simulink library "FlexBeamElement_MS2G_Lib"  (R2016a)
settings: Solver=ode45  StartTime=0.0  StopTime=10.0  RelTol=1e-3
undefined symbols (not defined in the file): b, beam_length, beam_wall, beam_width, bending_stiffness, Damping, density, Extr_Data_Box, kbendingx, kbendingy, kelongz, ktwistz, matDamping, num_elem, numelem, rho, shearM, X, Y, youngsM, Z
libraries: sm_lib x335, nesl_utility x64, FlexBeamElement_MS2G_Lib x1
(part 1 of 10)
Description:
  | Copyright 2014-2016 The MathWorks, Inc.
settings Model: Creator=psanghvi  LastModifiedBy=smiller
settings DataIOCC: LimitDataPoints=on  SaveFormat=Array  SignalLoggingSaveFormat=ModelDataLogs
settings DebuggingCC: UnderspecifiedInitializationDetection=Classic  MergeDetectMultiDrivingBlocksExec=none  SolverPrmCheckMsg=warning  MultiTaskDSMMsg=warning  MultiTaskCondExecSysMsg=none  AllowSymbolicDim=off
settings HardwareCC: ProdBitPerPointer=32  ProdLargestAtomicFloat=None  ProdIntDivRoundTo=Undefined  ProdEndianess=Unspecified  ProdWordSize=32  ProdHWDeviceType=32-bit Generic
settings ModelReferenceCC: PropagateSignalLabelsOutOfModel=off
settings ConfigComp: CovModelRefEnable=Off  CovSFcnEnable=off

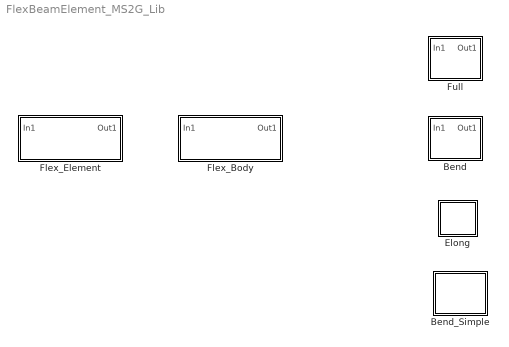
== system FlexBeamElement_MS2G_Lib ==
  Bend : Subsystem  mask{length=length, rho=rho, beam_width=beam_width, beam_wall=beam_wall, kbendingx=kbendingx, kbendingy=kbendingy, kbendingz=ktwistz, kelongz=kelongz, b=b}
      mask prompts: length "Beam Length (m)"; rho "Material Density (kg/(m^3)"; beam_width "Beam Width & Height (m)"; beam_wall "Beam Wall Thickness (m)"; kbendingx "Bending Spring Constant about X(Nm/rad)"; kbendingy "Bending Spring Constant about Y(Nm/rad)"; kbendingz "Twist Spring Constant about Z(Nm/rad)"; kelongz "Elongation Spring Constant about Z(N/m)"; b "Damping Constant (Nm/rad.s)"
  Bend_Simple : Subsystem  mask{length=length, rho=rho, beam_width=beam_width, beam_wall=beam_wall, kbendingx=kbendingx, kbendingy=kbendingy, kbendingz=ktwistz, kelongz=kelongz, b=b}
      mask prompts: length "Beam Length (m)"; rho "Material Density (kg/(m^3)"; beam_width "Beam Width & Height (m)"; beam_wall "Beam Wall Thickness (m)"; kbendingx "Bending Spring Constant about X(Nm/rad)"; kbendingy "Bending Spring Constant about Y(Nm/rad)"; kbendingz "Twist Spring Constant about Z(Nm/rad)"; kelongz "Elongation Spring Constant about Z(N/m)"; b "Damping Constant (Nm/rad.s)"
  Elong : Subsystem  mask{length=beam_length, kBending=bending_stiffness, matDamping=matDamping, beam_width=beam_width, beam_wall=beam_wall, rho=density}
      mask prompts: length "Beam Length (m)"; kBending "Bending Stiffness (N*m/rad)"; matDamping "Material Damping (N*m/(rad/s))"; beam_width "Beam Width & Height (m)"; beam_wall "Beam Wall Thickness(m)"; rho "Material Density (kg/(m^3)"
  Flex_Body : Subsystem  mask(Flexible Body){rho=density, youngsM=youngsM, shearM=shearM, numelem=num_elem, beam_length=beam_length, beam_width=beam_width, beam_wall=beam_wall, b=Damping}
      mask prompts: rho "Material Density (kg/(m^3)"; youngsM "Modulus of Elasticity (N/m2)"; shearM "Shear Modulus (N/m2)"; numelem "Number of elements"; beam_length "Beam Length (m)"; beam_width "Beam Width & Height (m)"; beam_wall "Beam Wall Thickness(m)"; b "Damping Constant (Nm/rad.s)"
      mask help:
      | Models a flexible hollow square beam based on lumped parameter method.
      | Number of flexible elements, material properties as well as beam
      | dimension can be varied from mask parameters.
      mask init:
      | [kbendingx, kbendingy, ktwistz, kelongz, length] = Compute_GFE_Prop(rho, youngsM, shearM, numelem, beam_length, beam_width,beam_wall);
      | thisblock = gcb;
      | anno = ['No of Elem: ' num2str(numelem)];
      | set_param(thisblock, 'AttributesFormatString',anno);
      | set_param([thisblock '/Matrix Concatenate'],'NumInputs','numelem')
      | blkchoice = get_param('FlexBeamElement_MS2G_Lib/Flex_Element','BlockChoice');
      | if numelem <1
      |     error('Number of Flexible elements should be greater than 0')
      | end
      | prev_flex_bod = find_system(gcb,'LookUnderMasks','all','RegExp','on','Name','Flex_Elem_*');
      | if ~isempty(prev_flex_bod)
      |     delete_block(prev_flex_bod(1:end))
      | end
      | linehan = find_system(thisblock,'LookUnderMasks','all','FindAll','on','type','line');
      | if ~isempty(linehan)
      |     delete_line(linehan)
      | end
      | blk_or = [100 155 140 195];
      | set_param([thisblock '/B'],'Position',blk_or)
      | set_param([thisblock '/' sprintf('Transform\nBeamX')],'Position',blk_or+[80 0 80 0])
      | add_line(thisblock,['B/Rconn1'],[sprintf('Transform\nBeamX') '/Lconn1'],'autorouting','on');
      | add_block('FlexBeamElement_MS2G_Lib/Flex_Element',[thisblock '/Flex_Elem_' num2str(1)],'Position',blk_or+[80 0 80 0]*2)
      | add_line(thisblock,[sprintf('Transform\nBeamX') '/Rconn1'],['Flex_Elem_' num2str(1) '/Lconn1'],'autorouting','on');
      | add_line(thisblock,'In1/1',['Flex_Elem_' num2str(1) '/1'],'autorouting','on')
      | add_line(thisblock,['Flex_Elem_' num2str(1) '/1'],'Matrix Concatenate/1','autorouting','on')
      | set_param([thisblock '/Flex_Elem_' num2str(1)], 'LinkStatus', 'none')
      | set_param([thisblock '/Flex_Elem_' num2str(1) '/' blkchoice], 'LinkStatus', 'none')
      | set_param([thisblock '/Flex_Elem_' num2str(1) '/' blkchoice '/Selector'],'InputPortWidth','3*numelem')
      | set_param([thisblock '/Flex_Elem_' num2str(1) '/' blkchoice '/Selector'],'Indices','[1 2 3]')
      | if strcmp(blkchoice,'Full')
      |     state_order{1} = [thisblock '/Flex_Elem_' num2str(1) '/' blkchoice '/Bearing Joint'];
      | elseif strcmp(blkchoice,'Elong')
      |     state_order{1} = [thisblock '/Flex_Elem_' num2str(1) '/' blkchoice '/Prismatic Joint'];
      | else
      |     state_order{1} = [thisblock '/Flex_Elem_' num2str(1) '/' blkchoice '/Revolute Joint'];
      | end
      | for i = 2:1:numelem
      |     add_block('FlexBeamElement_MS2G_Lib/Flex_Element',[thisblock '/Flex_Elem_' num2str(i)],'Position',blk_or+(i+1)*[80 0 80 0])
      |     add_line(thisblock,['Flex_Elem_' num2str(i-1) '/Rconn1'],['Flex_Elem_' num2str(i) '/Lconn1'],'autorouting','on');
      |     add_line(thisblock,'In1/1',['Flex_Elem_' num2str(i) '/1'],'autorouting','on')
      |     add_line(thisblock,['Flex_Elem_' num2str(i) '/1'],['Matrix Concatenate/' num2str(i)],'autorouting','on')
      |     set_param([thisblock '/Flex_Elem_' num2str(i)], 'LinkStatus', 'none')
      |     set_param([thisblock '/Flex_Elem_' num2str(i) '/' blkchoice], 'LinkStatus', 'none')
      |     set_param([thisblock '/Flex_Elem_' num2str(i) '/' blkchoice '/Selector'],'InputPortWidth','3*numelem')
      |     set_param([thisblock '/Flex_Elem_' num2str(i) '/' blkchoice '/Selector'],'Indices',['[' num2str([3*i-2 3*i-1 3*i]) ']'])
      |     if strcmp(blkchoice,'Full')
      |         state_order{i} = [thisblock '/Flex_Elem_' num2str(i) '/' blkchoice '/Bearing Joint'];
      |     elseif strcmp(blkchoice,'Elong')
      |         state_order{i} = [thisblock '/Flex_Elem_' num2str(i) '/' blkchoice '/Prismatic Joint'];
      |     else
      |         state_order{i} = [thisblock '/Flex_Elem_' num2str(i) '/' blkchoice '/Revolute Joint'];
      |     end
      | end
      | set_param([thisblock '/F'],'Position',blk_or+ (numelem+2)*[80 0 80 0]);
      | add_line(thisblock,['Flex_Elem_' num2str(numelem) '/Rconn1'],['F/Rconn1'],'autorouting','on');
      | assignin('base','State_order',state_order)
      | add_line(thisblock,'Matrix Concatenate/1','Out1/1','autorouting','on')
      settings: AttributesFormatString=No of Elem: 30  CopyFcn=set_param(gcb, 'LinkStatus', 'none')
      mask Display:
      | image(imread('Flexible_Beam.png'));
      | port_label('input',1,'F_L');
      | port_label('output',1,'wz');
      | color red
      | port_label('LConn',1,'B');
      | port_label('RConn',1,'F');
  Flex_Element : Subsystem  BlockChoice=Full
      settings: TemplateBlock=self  MemberBlocks=Bend,Elong,Full
  Full : Subsystem  mask{length=length, rho=rho, beam_width=beam_width, beam_wall=beam_wall, kbendingx=kbendingx, kbendingy=kbendingy, kbendingz=ktwistz, kelongz=kelongz, b=b}
      mask prompts: length "Beam Length (m)"; rho "Material Density (kg/(m^3)"; beam_width "Beam Width & Height (m)"; beam_wall "Beam Wall Thickness (m)"; kbendingx "Bending Spring Constant about X(Nm/rad)"; kbendingy "Bending Spring Constant about Y(Nm/rad)"; kbendingz "Twist Spring Constant about Z(Nm/rad)"; kelongz "Elongation Spring Constant about Z(N/m)"; b "Damping Constant (Nm/rad.s)"

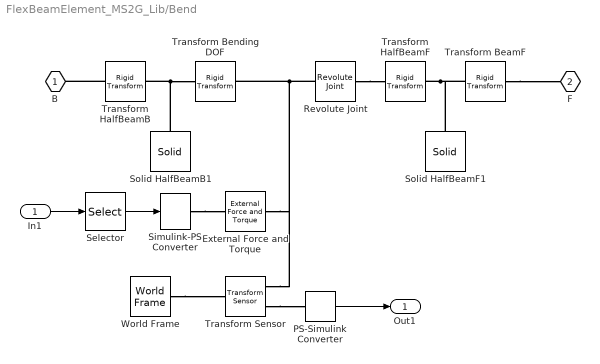
== system FlexBeamElement_MS2G_Lib/Bend ==
  In1 : Inport
  " Transform Bending DOF" : sm_lib/Frames and Transforms/Rigid Transform  TranslationMethod=StandardAxis  TranslationLengthUnit=m  TranslationStandardAxis=+Z  TranslationStandardOffset=length/4  TranslationCartesianOffset=[0 0 0]  TranslationROffset=0  TranslationROffsetUnits=m  TranslationZOffset=0  TranslationZOffsetUnits=m  TranslationThetaOffset=0  TranslationThetaOffsetUnits=deg  RotationMethod=StandardAxis  RotationAngleUnits=deg  RotationStandardAxis=+Y  RotationAngle=90  RotationArbitraryAxis=[0 0 1]  FollAlignAxisA=+X  BaseAlignAxisA=+Y  FollAlignAxisB=+Y  BaseAlignAxisB=+Z  RotationSequenceAxes=FollowerAxes  RotationSequence=XYX  RotationSequenceAngles=[0 0 0]  RotationSequenceAnglesUnits=deg  RotationMatrix=[1 0 0; 0 1 0; 0 0 1]
  " Transform BeamF" : sm_lib/Frames and Transforms/Rigid Transform  TranslationMethod=StandardAxis  TranslationLengthUnit=m  TranslationStandardAxis=+Z  TranslationStandardOffset=length/4  TranslationCartesianOffset=[0 0 0]  TranslationROffset=0  TranslationROffsetUnits=m  TranslationZOffset=0  TranslationZOffsetUnits=m  TranslationThetaOffset=0  TranslationThetaOffsetUnits=deg  RotationMethod=None  RotationAngleUnits=deg  RotationStandardAxis=+Z  RotationAngle=0  RotationArbitraryAxis=[0 0 1]  FollAlignAxisA=+X  BaseAlignAxisA=+Y  FollAlignAxisB=+Y  BaseAlignAxisB=+Z  RotationSequenceAxes=FollowerAxes  RotationSequence=XYX  RotationSequenceAngles=[0 0 0]  RotationSequenceAnglesUnits=deg  RotationMatrix=[1 0 0; 0 1 0; 0 0 1]
  External Force and Torque : sm_lib/Forces and Torques/External Force and Torque  ForceResolutionFrame=AttachedFrame  EnableForceX=off  EnableForceY=off  EnableForceZ=off  EnableForce=on  TorqueResolutionFrame=AttachedFrame  EnableTorqueX=off  EnableTorqueY=off  EnableTorqueZ=off  EnableTorque=off
  PS-Simulink Converter : nesl_utility/PS-Simulink Converter  PhysicalDomain=network_engine_domain  SubClassName=ps_output  LeftPortType=input  RightPortType=output  PseudoPeriodic=off  Frequencies=[]  Unit=1  AffineConversion=off
  Revolute Joint : sm_lib/Joints/Revolute Joint  SenseConstraintForce=off  SenseConstraintForceX=off  SenseConstraintForceY=off  SenseConstraintForceZ=off  SenseConstraintTorque=off  SenseConstraintTorqueX=off  SenseConstraintTorqueY=off  SenseConstraintTorqueZ=off  SenseTotalForce=off  SenseTotalForceX=off  SenseTotalForceY=off  SenseTotalForceZ=off  SenseTotalTorque=off  SenseTotalTorqueX=off  SenseTotalTorqueY=off  SenseTotalTorqueZ=off  CompositeWrenchDir=FollowerOnBase  CompositeWrenchFrame=BaseFrame  EquilibriumPosition=0  EquilibriumPositionUnits=deg  SpringStiffness=kbendingx  SpringStiffnessUnits=N*m/rad  DampingCoefficient=b  DampingCoefficientUnits=N*m/(rad/s)  TorqueActuationMode=NoTorque  MotionActuationMode=ComputedMotion  SensePosition=off  SenseVelocity=off  SenseAcceleration=off  SenseTorqueForce=off  PositionTargetSpecify=off  PositionTargetPriority=High  PositionTargetValue=0  PositionTargetValueUnits=deg  VelocityTargetSpecify=off  VelocityTargetPriority=High  VelocityTargetValue=0  VelocityTargetValueUnits=deg/s
  Selector : Selector  InputPortWidth=numelem*3  IndexOptions=Index vector (dialog)  Indices=[1 3]  OutputSizes=1
  Simulink-PS Converter : nesl_utility/Simulink-PS Converter  PhysicalDomain=network_engine_domain  SubClassName=ps_input  LeftPortType=input  RightPortType=output  PseudoPeriodic=off  Frequencies=[]  NoiseDistribution=none  NoiseParameters=[]  Unit=1  AffineConversion=off  InputFiltering=off  SimscapeFilterOrder=1  InputFilterTimeConstant=0.001  UdotUserProvided=1
  Solid HalfBeamB1 : sm_lib/Body Elements/Solid  InertiaType=CalculateFromGeometry  Mass=1  MassUnits=kg  CenterOfMass=[0 0 0]  CenterOfMassUnits=m  MomentsOfInertia=[1 1 1]  MomentsOfInertiaUnits=kg*m^2  ProductsOfInertia=[0 0 0]  ProductsOfInertiaUnits=kg*m^2  DensityBased=on  Density=rho  DensityUnits=kg/(m^3)  DoExposeReferenceFrame=on  SerializedFrames=<Frames/>  GraphicType=FromGeometry  MarkerShape=Sphere  MarkerSize=10  MarkerSizeUnits=m  GraphicVisPropType=SimpleVisualProperties  GraphicDiffuseColor=[0.5 0.5 0.5]  GraphicSpecularColor=[0.5 0.5 0.5 1.0]  GraphicAmbientColor=[0.15 0.15 0.15 1.0]  GraphicEmissiveColor=[0.0 0.0 0.0 1.0]  GraphicShininess=75  GraphicOpacity=1.0  GeometryShape=GeneralExtrusion  RectangleSize=[1 1]  RectangleSizeUnits=m  BrickDimensions=[1 1 1]  BrickDimensionUnits=m  CylinderRadius=1  CylinderRadiusUnits=m  CylinderLength=1  CylinderLengthUnits=m  SphereRadius=1  SphereRadiusUnits=m  EllipsoidRadii=[1 1 1]  EllipsoidRadiiUnits=m  ExtrusionCrossSection=Extr_Data_Box(beam_width,beam_width-2*beam_wall,beam_width,beam_width-2*beam_wall)  ExtrusionCrossSectionUnits=m  ExtrusionLength=length/2  ExtrusionLengthUnits=m  PolygonNumSides=3  PolygonOuterRadius=1  PolygonOuterRadiusUnits=m  ExtGeomFileType=STL  ExtGeomFileUnits=m  RevolutionCrossSection=[1 1; 1 -1; 2 -1; 2 1]  RevolutionCrossSectionUnits=m  RevolutionExtent=Full  RevolutionAngle=180  RevolutionAngleUnits=deg
  Solid HalfBeamF1 : sm_lib/Body Elements/Solid  InertiaType=CalculateFromGeometry  Mass=1  MassUnits=kg  CenterOfMass=[0 0 0]  CenterOfMassUnits=m  MomentsOfInertia=[1 1 1]  MomentsOfInertiaUnits=kg*m^2  ProductsOfInertia=[0 0 0]  ProductsOfInertiaUnits=kg*m^2  DensityBased=on  Density=rho  DensityUnits=kg/(m^3)  DoExposeReferenceFrame=on  SerializedFrames=<Frames/>  GraphicType=FromGeometry  MarkerShape=Sphere  MarkerSize=10  MarkerSizeUnits=m  GraphicVisPropType=SimpleVisualProperties  GraphicDiffuseColor=[0.5 0.5 0.5]  GraphicSpecularColor=[0.5 0.5 0.5 1.0]  GraphicAmbientColor=[0.15 0.15 0.15 1.0]  GraphicEmissiveColor=[0.0 0.0 0.0 1.0]  GraphicShininess=75  GraphicOpacity=1.0  GeometryShape=GeneralExtrusion  RectangleSize=[1 1]  RectangleSizeUnits=m  BrickDimensions=[1 1 1]  BrickDimensionUnits=m  CylinderRadius=1  CylinderRadiusUnits=m  CylinderLength=1  CylinderLengthUnits=m  SphereRadius=1  SphereRadiusUnits=m  EllipsoidRadii=[1 1 1]  EllipsoidRadiiUnits=m  ExtrusionCrossSection=Extr_Data_Box(beam_width,beam_width-2*beam_wall,beam_width,beam_width-2*beam_wall)  ExtrusionCrossSectionUnits=m  ExtrusionLength=length/2  ExtrusionLengthUnits=m  PolygonNumSides=3  PolygonOuterRadius=1  PolygonOuterRadiusUnits=m  ExtGeomFileType=STL  ExtGeomFileUnits=m  RevolutionCrossSection=[1 1; 1 -1; 2 -1; 2 1]  RevolutionCrossSectionUnits=m  RevolutionExtent=Full  RevolutionAngle=180  RevolutionAngleUnits=deg
  Transform HalfBeamB : sm_lib/Frames and Transforms/Rigid Transform  TranslationMethod=StandardAxis  TranslationLengthUnit=m  TranslationStandardAxis=+Z  TranslationStandardOffset=length/4  TranslationCartesianOffset=[0 0 0]  TranslationROffset=0  TranslationROffsetUnits=m  TranslationZOffset=0  TranslationZOffsetUnits=m  TranslationThetaOffset=0  TranslationThetaOffsetUnits=deg  RotationMethod=None  RotationAngleUnits=deg  RotationStandardAxis=+Z  RotationAngle=0  RotationArbitraryAxis=[0 0 1]  FollAlignAxisA=+X  BaseAlignAxisA=+Y  FollAlignAxisB=+Y  BaseAlignAxisB=+Z  RotationSequenceAxes=FollowerAxes  RotationSequence=XYX  RotationSequenceAngles=[0 0 0]  RotationSequenceAnglesUnits=deg  RotationMatrix=[1 0 0; 0 1 0; 0 0 1]
  Transform HalfBeamF : sm_lib/Frames and Transforms/Rigid Transform  TranslationMethod=StandardAxis  TranslationLengthUnit=m  TranslationStandardAxis=+Z  TranslationStandardOffset=-length/4  TranslationCartesianOffset=[0 0 0]  TranslationROffset=0  TranslationROffsetUnits=m  TranslationZOffset=0  TranslationZOffsetUnits=m  TranslationThetaOffset=0  TranslationThetaOffsetUnits=deg  RotationMethod=StandardAxis  RotationAngleUnits=deg  RotationStandardAxis=+Y  RotationAngle=90  RotationArbitraryAxis=[0 0 1]  FollAlignAxisA=+X  BaseAlignAxisA=+Y  FollAlignAxisB=+Y  BaseAlignAxisB=+Z  RotationSequenceAxes=FollowerAxes  RotationSequence=XYX  RotationSequenceAngles=[0 0 0]  RotationSequenceAnglesUnits=deg  RotationMatrix=[1 0 0; 0 1 0; 0 0 1]
  Transform Sensor : sm_lib/Frames and Transforms/Transform Sensor  MeasurementFrame=World  SenseAngle=off  SenseAxis=off  SenseAngle1=off  SenseAngle2=off  SenseAngle3=off  SenseQ=off  SenseR=off  SenseOmegaX=off  SenseOmegaY=off  SenseOmegaZ=on  SenseOmega1=off  SenseOmega2=off  SenseOmega3=off  SenseQDot=off  SenseRDot=off  SenseAlphaX=off  SenseAlphaY=off  SenseAlphaZ=off  SenseAlpha1=off  SenseAlpha2=off  SenseAlpha3=off  SenseQDDot=off  SenseRDDot=off  SenseX=off  SenseY=off  SenseZ=off  SenseRad=off  SenseAzim=off  SenseDist=off  SenseInc=off  SenseXDot=off  SenseYDot=off  SenseZDot=off  SenseRadDot=off  SenseAzimDot=off  SenseDistDot=off  SenseIncDot=off  SenseXDDot=off  SenseYDDot=off  SenseZDDot=off  SenseRadDDot=off  SenseAzimDDot=off  SenseDistDDot=off  SenseIncDDot=off
  World Frame : sm_lib/Frames and Transforms/World Frame
  B : PMIOPort  Port=1  Side=Left
  F : PMIOPort  Port=2  Side=Right
  Out1 : Outport
  wires:
  In1/1 -> Selector/1
  Selector/1 -> Simulink-PS Converter/1
  PS-Simulink Converter/1 -> Out1/1
  connections:
  " Transform BeamF"/RConn1 -- F/RConn1
  Transform HalfBeamB/LConn1 -- B/RConn1
  Transform HalfBeamF/LConn1 -- " Transform BeamF"/LConn1 -- Solid HalfBeamF1/RConn1
  Solid HalfBeamB1/RConn1 -- Transform HalfBeamB/RConn1 -- " Transform Bending DOF"/LConn1
  Revolute Joint/RConn1 -- Transform HalfBeamF/RConn1
  Revolute Joint/LConn1 -- Transform Sensor/RConn1 -- External Force and Torque/RConn1 -- " Transform Bending DOF"/RConn1
  Simulink-PS Converter/RConn1 -- External Force and Torque/LConn1
  World Frame/RConn1 -- Transform Sensor/LConn1
  Transform Sensor/RConn2 -- PS-Simulink Converter/LConn1

== system FlexBeamElement_MS2G_Lib/Bend_Simple ==
  " Transform BeamF" : sm_lib/Frames and Transforms/Rigid Transform  TranslationMethod=StandardAxis  TranslationLengthUnit=m  TranslationStandardAxis=+Z  TranslationStandardOffset=length/4  TranslationCartesianOffset=[0 0 0]  TranslationROffset=0  TranslationROffsetUnits=m  TranslationZOffset=0  TranslationZOffsetUnits=m  TranslationThetaOffset=0  TranslationThetaOffsetUnits=deg  RotationMethod=None  RotationAngleUnits=deg  RotationStandardAxis=+Z  RotationAngle=0  RotationArbitraryAxis=[0 0 1]  FollAlignAxisA=+X  BaseAlignAxisA=+Y  FollAlignAxisB=+Y  BaseAlignAxisB=+Z  RotationSequenceAxes=FollowerAxes  RotationSequence=XYX  RotationSequenceAngles=[0 0 0]  RotationSequenceAnglesUnits=deg  RotationMatrix=[1 0 0; 0 1 0; 0 0 1]
  " Transform Bending DOF" : sm_lib/Frames and Transforms/Rigid Transform  TranslationMethod=StandardAxis  TranslationLengthUnit=m  TranslationStandardAxis=+Z  TranslationStandardOffset=length/4  TranslationCartesianOffset=[0 0 0]  TranslationROffset=0  TranslationROffsetUnits=m  TranslationZOffset=0  TranslationZOffsetUnits=m  TranslationThetaOffset=0  TranslationThetaOffsetUnits=deg  RotationMethod=StandardAxis  RotationAngleUnits=deg  RotationStandardAxis=+Y  RotationAngle=90  RotationArbitraryAxis=[0 0 1]  FollAlignAxisA=+X  BaseAlignAxisA=+Y  FollAlignAxisB=+Y  BaseAlignAxisB=+Z  RotationSequenceAxes=FollowerAxes  RotationSequence=XYX  RotationSequenceAngles=[0 0 0]  RotationSequenceAnglesUnits=deg  RotationMatrix=[1 0 0; 0 1 0; 0 0 1]
  Revolute Joint : sm_lib/Joints/Revolute Joint  SenseConstraintForce=off  SenseConstraintForceX=off  SenseConstraintForceY=off  SenseConstraintForceZ=off  SenseConstraintTorque=off  SenseConstraintTorqueX=off  SenseConstraintTorqueY=off  SenseConstraintTorqueZ=off  SenseTotalForce=off  SenseTotalForceX=off  SenseTotalForceY=off  SenseTotalForceZ=off  SenseTotalTorque=off  SenseTotalTorqueX=off  SenseTotalTorqueY=off  SenseTotalTorqueZ=off  CompositeWrenchDir=FollowerOnBase  CompositeWrenchFrame=BaseFrame  EquilibriumPosition=0  EquilibriumPositionUnits=deg  SpringStiffness=kbendingx  SpringStiffnessUnits=N*m/rad  DampingCoefficient=b  DampingCoefficientUnits=N*m/(rad/s)  TorqueActuationMode=NoTorque  MotionActuationMode=ComputedMotion  SensePosition=off  SenseVelocity=off  SenseAcceleration=off  SenseTorqueForce=off  PositionTargetSpecify=off  PositionTargetPriority=High  PositionTargetValue=0  PositionTargetValueUnits=deg  VelocityTargetSpecify=off  VelocityTargetPriority=High  VelocityTargetValue=0  VelocityTargetValueUnits=deg/s
  Solid HalfBeamB1 : sm_lib/Body Elements/Solid  InertiaType=CalculateFromGeometry  Mass=1  MassUnits=kg  CenterOfMass=[0 0 0]  CenterOfMassUnits=m  MomentsOfInertia=[1 1 1]  MomentsOfInertiaUnits=kg*m^2  ProductsOfInertia=[0 0 0]  ProductsOfInertiaUnits=kg*m^2  DensityBased=on  Density=rho  DensityUnits=kg/(m^3)  DoExposeReferenceFrame=on  SerializedFrames=<Frames/>  GraphicType=FromGeometry  MarkerShape=Sphere  MarkerSize=10  MarkerSizeUnits=m  GraphicVisPropType=SimpleVisualProperties  GraphicDiffuseColor=[0.5 0.5 0.5]  GraphicSpecularColor=[0.5 0.5 0.5 1.0]  GraphicAmbientColor=[0.15 0.15 0.15 1.0]  GraphicEmissiveColor=[0.0 0.0 0.0 1.0]  GraphicShininess=75  GraphicOpacity=1.0  GeometryShape=GeneralExtrusion  RectangleSize=[1 1]  RectangleSizeUnits=m  BrickDimensions=[1 1 1]  BrickDimensionUnits=m  CylinderRadius=1  CylinderRadiusUnits=m  CylinderLength=1  CylinderLengthUnits=m  SphereRadius=1  SphereRadiusUnits=m  EllipsoidRadii=[1 1 1]  EllipsoidRadiiUnits=m  ExtrusionCrossSection=Extr_Data_Box(beam_width,beam_width-2*beam_wall,beam_width,beam_width-2*beam_wall)  ExtrusionCrossSectionUnits=m  ExtrusionLength=length/2  ExtrusionLengthUnits=m  PolygonNumSides=3  PolygonOuterRadius=1  PolygonOuterRadiusUnits=m  ExtGeomFileType=STL  ExtGeomFileUnits=m  RevolutionCrossSection=[1 1; 1 -1; 2 -1; 2 1]  RevolutionCrossSectionUnits=m  RevolutionExtent=Full  RevolutionAngle=180  RevolutionAngleUnits=deg
  Solid HalfBeamF1 : sm_lib/Body Elements/Solid  InertiaType=CalculateFromGeometry  Mass=1  MassUnits=kg  CenterOfMass=[0 0 0]  CenterOfMassUnits=m  MomentsOfInertia=[1 1 1]  MomentsOfInertiaUnits=kg*m^2  ProductsOfInertia=[0 0 0]  ProductsOfInertiaUnits=kg*m^2  DensityBased=on  Density=rho  DensityUnits=kg/(m^3)  DoExposeReferenceFrame=on  SerializedFrames=<Frames/>  GraphicType=FromGeometry  MarkerShape=Sphere  MarkerSize=10  MarkerSizeUnits=m  GraphicVisPropType=SimpleVisualProperties  GraphicDiffuseColor=[0.5 0.5 0.5]  GraphicSpecularColor=[0.5 0.5 0.5 1.0]  GraphicAmbientColor=[0.15 0.15 0.15 1.0]  GraphicEmissiveColor=[0.0 0.0 0.0 1.0]  GraphicShininess=75  GraphicOpacity=1.0  GeometryShape=GeneralExtrusion  RectangleSize=[1 1]  RectangleSizeUnits=m  BrickDimensions=[1 1 1]  BrickDimensionUnits=m  CylinderRadius=1  CylinderRadiusUnits=m  CylinderLength=1  CylinderLengthUnits=m  SphereRadius=1  SphereRadiusUnits=m  EllipsoidRadii=[1 1 1]  EllipsoidRadiiUnits=m  ExtrusionCrossSection=Extr_Data_Box(beam_width,beam_width-2*beam_wall,beam_width,beam_width-2*beam_wall)  ExtrusionCrossSectionUnits=m  ExtrusionLength=length/2  ExtrusionLengthUnits=m  PolygonNumSides=3  PolygonOuterRadius=1  PolygonOuterRadiusUnits=m  ExtGeomFileType=STL  ExtGeomFileUnits=m  RevolutionCrossSection=[1 1; 1 -1; 2 -1; 2 1]  RevolutionCrossSectionUnits=m  RevolutionExtent=Full  RevolutionAngle=180  RevolutionAngleUnits=deg
  Transform HalfBeamB : sm_lib/Frames and Transforms/Rigid Transform  TranslationMethod=StandardAxis  TranslationLengthUnit=m  TranslationStandardAxis=+Z  TranslationStandardOffset=length/4  TranslationCartesianOffset=[0 0 0]  TranslationROffset=0  TranslationROffsetUnits=m  TranslationZOffset=0  TranslationZOffsetUnits=m  TranslationThetaOffset=0  TranslationThetaOffsetUnits=deg  RotationMethod=None  RotationAngleUnits=deg  RotationStandardAxis=+Z  RotationAngle=0  RotationArbitraryAxis=[0 0 1]  FollAlignAxisA=+X  BaseAlignAxisA=+Y  FollAlignAxisB=+Y  BaseAlignAxisB=+Z  RotationSequenceAxes=FollowerAxes  RotationSequence=XYX  RotationSequenceAngles=[0 0 0]  RotationSequenceAnglesUnits=deg  RotationMatrix=[1 0 0; 0 1 0; 0 0 1]
  Transform HalfBeamF : sm_lib/Frames and Transforms/Rigid Transform  TranslationMethod=StandardAxis  TranslationLengthUnit=m  TranslationStandardAxis=+Z  TranslationStandardOffset=-length/4  TranslationCartesianOffset=[0 0 0]  TranslationROffset=0  TranslationROffsetUnits=m  TranslationZOffset=0  TranslationZOffsetUnits=m  TranslationThetaOffset=0  TranslationThetaOffsetUnits=deg  RotationMethod=StandardAxis  RotationAngleUnits=deg  RotationStandardAxis=+Y  RotationAngle=90  RotationArbitraryAxis=[0 0 1]  FollAlignAxisA=+X  BaseAlignAxisA=+Y  FollAlignAxisB=+Y  BaseAlignAxisB=+Z  RotationSequenceAxes=FollowerAxes  RotationSequence=XYX  RotationSequenceAngles=[0 0 0]  RotationSequenceAnglesUnits=deg  RotationMatrix=[1 0 0; 0 1 0; 0 0 1]
  B : PMIOPort  Port=1  Side=Left
  F : PMIOPort  Port=2  Side=Right
  connections:
  Revolute Joint/LConn1 -- " Transform Bending DOF"/RConn1
  Revolute Joint/RConn1 -- Transform HalfBeamF/RConn1
  " Transform Bending DOF"/LConn1 -- Transform HalfBeamB/RConn1 -- Solid HalfBeamB1/RConn1
  Solid HalfBeamF1/RConn1 -- " Transform BeamF"/LConn1 -- Transform HalfBeamF/LConn1
  Transform HalfBeamB/LConn1 -- B/RConn1
  " Transform BeamF"/RConn1 -- F/RConn1

== system FlexBeamElement_MS2G_Lib/Elong ==
  " Transform Bending DOF" : sm_lib/Frames and Transforms/Rigid Transform  TranslationMethod=StandardAxis  TranslationLengthUnit=m  TranslationStandardAxis=+Z  TranslationStandardOffset=length/4  TranslationCartesianOffset=[0 0 0]  TranslationROffset=0  TranslationROffsetUnits=m  TranslationZOffset=0  TranslationZOffsetUnits=m  TranslationThetaOffset=0  TranslationThetaOffsetUnits=deg  RotationMethod=None  RotationAngleUnits=deg  RotationStandardAxis=+Y  RotationAngle=90  RotationArbitraryAxis=[0 0 1]  FollAlignAxisA=+X  BaseAlignAxisA=+Y  FollAlignAxisB=+Y  BaseAlignAxisB=+Z  RotationSequenceAxes=FollowerAxes  RotationSequence=XYX  RotationSequenceAngles=[0 0 0]  RotationSequenceAnglesUnits=deg  RotationMatrix=[1 0 0; 0 1 0; 0 0 1]
  " Transform BeamF" : sm_lib/Frames and Transforms/Rigid Transform  TranslationMethod=StandardAxis  TranslationLengthUnit=m  TranslationStandardAxis=+Z  TranslationStandardOffset=length/4  TranslationCartesianOffset=[0 0 0]  TranslationROffset=0  TranslationROffsetUnits=m  TranslationZOffset=0  TranslationZOffsetUnits=m  TranslationThetaOffset=0  TranslationThetaOffsetUnits=deg  RotationMethod=None  RotationAngleUnits=deg  RotationStandardAxis=+Z  RotationAngle=0  RotationArbitraryAxis=[0 0 1]  FollAlignAxisA=+X  BaseAlignAxisA=+Y  FollAlignAxisB=+Y  BaseAlignAxisB=+Z  RotationSequenceAxes=FollowerAxes  RotationSequence=XYX  RotationSequenceAngles=[0 0 0]  RotationSequenceAnglesUnits=deg  RotationMatrix=[1 0 0; 0 1 0; 0 0 1]
  Prismatic Joint : sm_lib/Joints/Prismatic Joint  SenseConstraintForce=off  SenseConstraintForceX=off  SenseConstraintForceY=off  SenseConstraintForceZ=off  SenseConstraintTorque=off  SenseConstraintTorqueX=off  SenseConstraintTorqueY=off  SenseConstraintTorqueZ=off  SenseTotalForce=off  SenseTotalForceX=off  SenseTotalForceY=off  SenseTotalForceZ=off  SenseTotalTorque=off  SenseTotalTorqueX=off  SenseTotalTorqueY=off  SenseTotalTorqueZ=off  CompositeWrenchDir=FollowerOnBase  CompositeWrenchFrame=BaseFrame  EquilibriumPosition=0  EquilibriumPositionUnits=m  SpringStiffness=0  SpringStiffnessUnits=N/m  DampingCoefficient=0  DampingCoefficientUnits=N/(m/s)  TorqueActuationMode=NoTorque  MotionActuationMode=ComputedMotion  SensePosition=off  SenseVelocity=off  SenseAcceleration=off  SenseTorqueForce=off  PositionTargetSpecify=off  PositionTargetPriority=High  PositionTargetValue=0  PositionTargetValueUnits=m  VelocityTargetSpecify=off  VelocityTargetPriority=High  VelocityTargetValue=0  VelocityTargetValueUnits=m/s
  Solid HalfBeamB : sm_lib/Body Elements/Solid  InertiaType=CalculateFromGeometry  Mass=1  MassUnits=kg  CenterOfMass=[0 0 0]  CenterOfMassUnits=m  MomentsOfInertia=[1 1 1]  MomentsOfInertiaUnits=kg*m^2  ProductsOfInertia=[0 0 0]  ProductsOfInertiaUnits=kg*m^2  DensityBased=on  Density=rho  DensityUnits=kg/(m^3)  DoExposeReferenceFrame=on  SerializedFrames=<Frames/>  GraphicType=FromGeometry  MarkerShape=Sphere  MarkerSize=10  MarkerSizeUnits=m  GraphicVisPropType=SimpleVisualProperties  GraphicDiffuseColor=[0.5 0.5 0.5]  GraphicSpecularColor=[0.5 0.5 0.5 1.0]  GraphicAmbientColor=[0.15 0.15 0.15 1.0]  GraphicEmissiveColor=[0.0 0.0 0.0 1.0]  GraphicShininess=75  GraphicOpacity=1.0  GeometryShape=GeneralExtrusion  RectangleSize=[1 1]  RectangleSizeUnits=m  BrickDimensions=[1 1 1]  BrickDimensionUnits=m  CylinderRadius=1  CylinderRadiusUnits=m  CylinderLength=1  CylinderLengthUnits=m  SphereRadius=1  SphereRadiusUnits=m  EllipsoidRadii=[1 1 1]  EllipsoidRadiiUnits=m  ExtrusionCrossSection=Extr_Data_Box(beam_width,beam_width-2*beam_wall,beam_width,beam_width-2*beam_wall)  ExtrusionCrossSectionUnits=m  ExtrusionLength=length/2  ExtrusionLengthUnits=m  PolygonNumSides=3  PolygonOuterRadius=1  PolygonOuterRadiusUnits=m  ExtGeomFileType=STL  ExtGeomFileUnits=m  RevolutionCrossSection=[1 1; 1 -1; 2 -1; 2 1]  RevolutionCrossSectionUnits=m  RevolutionExtent=Full  RevolutionAngle=180  RevolutionAngleUnits=deg
  Solid HalfBeamF : sm_lib/Body Elements/Solid  InertiaType=CalculateFromGeometry  Mass=1  MassUnits=kg  CenterOfMass=[0 0 0]  CenterOfMassUnits=m  MomentsOfInertia=[1 1 1]  MomentsOfInertiaUnits=kg*m^2  ProductsOfInertia=[0 0 0]  ProductsOfInertiaUnits=kg*m^2  DensityBased=on  Density=rho  DensityUnits=kg/(m^3)  DoExposeReferenceFrame=on  SerializedFrames=<Frames/>  GraphicType=FromGeometry  MarkerShape=Sphere  MarkerSize=10  MarkerSizeUnits=m  GraphicVisPropType=SimpleVisualProperties  GraphicDiffuseColor=[0.5 0.5 0.5]  GraphicSpecularColor=[0.5 0.5 0.5 1.0]  GraphicAmbientColor=[0.15 0.15 0.15 1.0]  GraphicEmissiveColor=[0.0 0.0 0.0 1.0]  GraphicShininess=75  GraphicOpacity=1.0  GeometryShape=GeneralExtrusion  RectangleSize=[1 1]  RectangleSizeUnits=m  BrickDimensions=[1 1 1]  BrickDimensionUnits=m  CylinderRadius=1  CylinderRadiusUnits=m  CylinderLength=1  CylinderLengthUnits=m  SphereRadius=1  SphereRadiusUnits=m  EllipsoidRadii=[1 1 1]  EllipsoidRadiiUnits=m  ExtrusionCrossSection=Extr_Data_Box(beam_width,beam_width-2*beam_wall,beam_width,beam_width-2*beam_wall)  ExtrusionCrossSectionUnits=m  ExtrusionLength=length/2  ExtrusionLengthUnits=m  PolygonNumSides=3  PolygonOuterRadius=1  PolygonOuterRadiusUnits=m  ExtGeomFileType=STL  ExtGeomFileUnits=m  RevolutionCrossSection=[1 1; 1 -1; 2 -1; 2 1]  RevolutionCrossSectionUnits=m  RevolutionExtent=Full  RevolutionAngle=180  RevolutionAngleUnits=deg
  Transform HalfBeamB : sm_lib/Frames and Transforms/Rigid Transform  TranslationMethod=StandardAxis  TranslationLengthUnit=m  TranslationStandardAxis=+Z  TranslationStandardOffset=length/4  TranslationCartesianOffset=[0 0 0]  TranslationROffset=0  TranslationROffsetUnits=m  TranslationZOffset=0  TranslationZOffsetUnits=m  TranslationThetaOffset=0  TranslationThetaOffsetUnits=deg  RotationMethod=None  RotationAngleUnits=deg  RotationStandardAxis=+Z  RotationAngle=0  RotationArbitraryAxis=[0 0 1]  FollAlignAxisA=+X  BaseAlignAxisA=+Y  FollAlignAxisB=+Y  BaseAlignAxisB=+Z  RotationSequenceAxes=FollowerAxes  RotationSequence=XYX  RotationSequenceAngles=[0 0 0]  RotationSequenceAnglesUnits=deg  RotationMatrix=[1 0 0; 0 1 0; 0 0 1]
  Transform HalfBeamF : sm_lib/Frames and Transforms/Rigid Transform  TranslationMethod=StandardAxis  TranslationLengthUnit=m  TranslationStandardAxis=+Z  TranslationStandardOffset=-length/4  TranslationCartesianOffset=[0 0 0]  TranslationROffset=0  TranslationROffsetUnits=m  TranslationZOffset=0  TranslationZOffsetUnits=m  TranslationThetaOffset=0  TranslationThetaOffsetUnits=deg  RotationMethod=None  RotationAngleUnits=deg  RotationStandardAxis=+Y  RotationAngle=90  RotationArbitraryAxis=[0 0 1]  FollAlignAxisA=+X  BaseAlignAxisA=+Y  FollAlignAxisB=+Y  BaseAlignAxisB=+Z  RotationSequenceAxes=FollowerAxes  RotationSequence=XYX  RotationSequenceAngles=[0 0 0]  RotationSequenceAnglesUnits=deg  RotationMatrix=[1 0 0; 0 1 0; 0 0 1]
  B : PMIOPort  Port=1  Side=Left
  F : PMIOPort  Port=2  Side=Right
  connections:
  B/RConn1 -- Transform HalfBeamB/LConn1
  " Transform BeamF"/RConn1 -- F/RConn1
  Prismatic Joint/LConn1 -- " Transform Bending DOF"/RConn1
  Prismatic Joint/RConn1 -- Transform HalfBeamF/RConn1
  " Transform BeamF"/LConn1 -- Solid HalfBeamF/RConn1 -- Transform HalfBeamF/LConn1
  Transform HalfBeamB/RConn1 -- " Transform Bending DOF"/LConn1 -- Solid HalfBeamB/RConn1

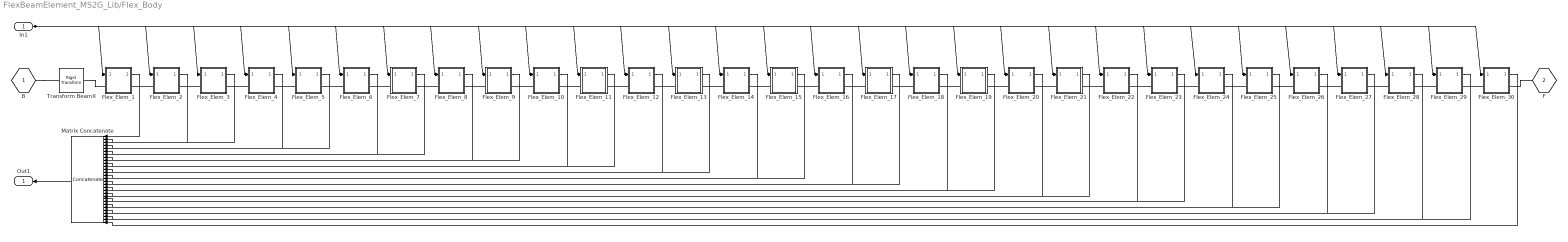
== system FlexBeamElement_MS2G_Lib/Flex_Body ==
  In1 : Inport
  Flex_Elem_1 : Subsystem  BlockChoice=Full
      settings: AttributesFormatString=%<BlockChoice>  TemplateBlock=FlexBeamElement_MS2G_Lib/Flex_Element  MemberBlocks=Bend,Elong,Full
  Flex_Elem_10 : Subsystem  BlockChoice=Full
      settings: AttributesFormatString=%<BlockChoice>  TemplateBlock=FlexBeamElement_MS2G_Lib/Flex_Element  MemberBlocks=Bend,Elong,Full
  Flex_Elem_11 : Subsystem  BlockChoice=Full
      settings: AttributesFormatString=%<BlockChoice>  TemplateBlock=FlexBeamElement_MS2G_Lib/Flex_Element  MemberBlocks=Bend,Elong,Full
  Flex_Elem_12 : Subsystem  BlockChoice=Full
      settings: AttributesFormatString=%<BlockChoice>  TemplateBlock=FlexBeamElement_MS2G_Lib/Flex_Element  MemberBlocks=Bend,Elong,Full
  Flex_Elem_13 : Subsystem  BlockChoice=Full
      settings: AttributesFormatString=%<BlockChoice>  TemplateBlock=FlexBeamElement_MS2G_Lib/Flex_Element  MemberBlocks=Bend,Elong,Full
  Flex_Elem_14 : Subsystem  BlockChoice=Full
      settings: AttributesFormatString=%<BlockChoice>  TemplateBlock=FlexBeamElement_MS2G_Lib/Flex_Element  MemberBlocks=Bend,Elong,Full
  Flex_Elem_15 : Subsystem  BlockChoice=Full
      settings: AttributesFormatString=%<BlockChoice>  TemplateBlock=FlexBeamElement_MS2G_Lib/Flex_Element  MemberBlocks=Bend,Elong,Full
  Flex_Elem_16 : Subsystem  BlockChoice=Full
      settings: AttributesFormatString=%<BlockChoice>  TemplateBlock=FlexBeamElement_MS2G_Lib/Flex_Element  MemberBlocks=Bend,Elong,Full
  Flex_Elem_17 : Subsystem  BlockChoice=Full
      settings: AttributesFormatString=%<BlockChoice>  TemplateBlock=FlexBeamElement_MS2G_Lib/Flex_Element  MemberBlocks=Bend,Elong,Full
  Flex_Elem_18 : Subsystem  BlockChoice=Full
      settings: AttributesFormatString=%<BlockChoice>  TemplateBlock=FlexBeamElement_MS2G_Lib/Flex_Element  MemberBlocks=Bend,Elong,Full
  Flex_Elem_19 : Subsystem  BlockChoice=Full
      settings: AttributesFormatString=%<BlockChoice>  TemplateBlock=FlexBeamElement_MS2G_Lib/Flex_Element  MemberBlocks=Bend,Elong,Full
  Flex_Elem_2 : Subsystem  BlockChoice=Full
      settings: AttributesFormatString=%<BlockChoice>  TemplateBlock=FlexBeamElement_MS2G_Lib/Flex_Element  MemberBlocks=Bend,Elong,Full
  Flex_Elem_20 : Subsystem  BlockChoice=Full
      settings: AttributesFormatString=%<BlockChoice>  TemplateBlock=FlexBeamElement_MS2G_Lib/Flex_Element  MemberBlocks=Bend,Elong,Full
  Flex_Elem_21 : Subsystem  BlockChoice=Full
      settings: AttributesFormatString=%<BlockChoice>  TemplateBlock=FlexBeamElement_MS2G_Lib/Flex_Element  MemberBlocks=Bend,Elong,Full
  Flex_Elem_22 : Subsystem  BlockChoice=Full
      settings: AttributesFormatString=%<BlockChoice>  TemplateBlock=FlexBeamElement_MS2G_Lib/Flex_Element  MemberBlocks=Bend,Elong,Full
  Flex_Elem_23 : Subsystem  BlockChoice=Full
      settings: AttributesFormatString=%<BlockChoice>  TemplateBlock=FlexBeamElement_MS2G_Lib/Flex_Element  MemberBlocks=Bend,Elong,Full
  Flex_Elem_24 : Subsystem  BlockChoice=Full
      settings: AttributesFormatString=%<BlockChoice>  TemplateBlock=FlexBeamElement_MS2G_Lib/Flex_Element  MemberBlocks=Bend,Elong,Full
  Flex_Elem_25 : Subsystem  BlockChoice=Full
      settings: AttributesFormatString=%<BlockChoice>  TemplateBlock=FlexBeamElement_MS2G_Lib/Flex_Element  MemberBlocks=Bend,Elong,Full
  Flex_Elem_26 : Subsystem  BlockChoice=Full
      settings: AttributesFormatString=%<BlockChoice>  TemplateBlock=FlexBeamElement_MS2G_Lib/Flex_Element  MemberBlocks=Bend,Elong,Full
  Flex_Elem_27 : Subsystem  BlockChoice=Full
      settings: AttributesFormatString=%<BlockChoice>  TemplateBlock=FlexBeamElement_MS2G_Lib/Flex_Element  MemberBlocks=Bend,Elong,Full
  Flex_Elem_28 : Subsystem  BlockChoice=Full
      settings: AttributesFormatString=%<BlockChoice>  TemplateBlock=FlexBeamElement_MS2G_Lib/Flex_Element  MemberBlocks=Bend,Elong,Full
  Flex_Elem_29 : Subsystem  BlockChoice=Full
      settings: AttributesFormatString=%<BlockChoice>  TemplateBlock=FlexBeamElement_MS2G_Lib/Flex_Element  MemberBlocks=Bend,Elong,Full
  Flex_Elem_3 : Subsystem  BlockChoice=Full
      settings: AttributesFormatString=%<BlockChoice>  TemplateBlock=FlexBeamElement_MS2G_Lib/Flex_Element  MemberBlocks=Bend,Elong,Full
  Flex_Elem_30 : Subsystem  BlockChoice=Full
      settings: AttributesFormatString=%<BlockChoice>  TemplateBlock=FlexBeamElement_MS2G_Lib/Flex_Element  MemberBlocks=Bend,Elong,Full
  Flex_Elem_4 : Subsystem  BlockChoice=Full
      settings: AttributesFormatString=%<BlockChoice>  TemplateBlock=FlexBeamElement_MS2G_Lib/Flex_Element  MemberBlocks=Bend,Elong,Full
  Flex_Elem_5 : Subsystem  BlockChoice=Full
      settings: AttributesFormatString=%<BlockChoice>  TemplateBlock=FlexBeamElement_MS2G_Lib/Flex_Element  MemberBlocks=Bend,Elong,Full
  Flex_Elem_6 : Subsystem  BlockChoice=Full
      settings: AttributesFormatString=%<BlockChoice>  TemplateBlock=FlexBeamElement_MS2G_Lib/Flex_Element  MemberBlocks=Bend,Elong,Full
  Flex_Elem_7 : Subsystem  BlockChoice=Full
      settings: AttributesFormatString=%<BlockChoice>  TemplateBlock=FlexBeamElement_MS2G_Lib/Flex_Element  MemberBlocks=Bend,Elong,Full
  Flex_Elem_8 : Subsystem  BlockChoice=Full
      settings: AttributesFormatString=%<BlockChoice>  TemplateBlock=FlexBeamElement_MS2G_Lib/Flex_Element  MemberBlocks=Bend,Elong,Full
  Flex_Elem_9 : Subsystem  BlockChoice=Full
      settings: AttributesFormatString=%<BlockChoice>  TemplateBlock=FlexBeamElement_MS2G_Lib/Flex_Element  MemberBlocks=Bend,Elong,Full
  Matrix Concatenate : Concatenate  NumInputs=numelem  Mode=Multidimensional array
  Transform BeamX : sm_lib/Frames and Transforms/Rigid Transform  TranslationMethod=StandardAxis  TranslationLengthUnit=m  TranslationStandardAxis=+Z  TranslationStandardOffset=0  TranslationCartesianOffset=[0 0 0]  TranslationROffset=0  TranslationROffsetUnits=m  TranslationZOffset=0  TranslationZOffsetUnits=m  TranslationThetaOffset=0  TranslationThetaOffsetUnits=deg  RotationMethod=StandardAxis  RotationAngleUnits=deg  RotationStandardAxis=+Y  RotationAngle=90  RotationArbitraryAxis=[0 0 1]  FollAlignAxisA=+X  BaseAlignAxisA=+Y  FollAlignAxisB=+Y  BaseAlignAxisB=+Z  RotationSequenceAxes=FollowerAxes  RotationSequence=XYX  RotationSequenceAngles=[0 0 0]  RotationSequenceAnglesUnits=deg  RotationMatrix=[1 0 0; 0 1 0; 0 0 1]
  B : PMIOPort  Port=1  Side=Left
  F : PMIOPort  Port=2  Side=Right
  Out1 : Outport
  wires:
  In1/1 -> Flex_Elem_1/1(In1), Flex_Elem_2/1(In1), Flex_Elem_3/1(In1), Flex_Elem_4/1(In1), Flex_Elem_5/1(In1), Flex_Elem_6/1(In1), Flex_Elem_7/1(In1), Flex_Elem_8/1(In1), Flex_Elem_9/1(In1), Flex_Elem_10/1(In1), Flex_Elem_11/1(In1), Flex_Elem_12/1(In1), Flex_Elem_13/1(In1), Flex_Elem_14/1(In1), Flex_Elem_15/1(In1), Flex_Elem_16/1(In1), Flex_Elem_17/1(In1), Flex_Elem_18/1(In1), Flex_Elem_19/1(In1), Flex_Elem_20/1(In1), Flex_Elem_21/1(In1), Flex_Elem_22/1(In1), Flex_Elem_23/1(In1), Flex_Elem_24/1(In1), Flex_Elem_25/1(In1), Flex_Elem_26/1(In1), Flex_Elem_27/1(In1), Flex_Elem_28/1(In1), Flex_Elem_29/1(In1), Flex_Elem_30/1(In1)
  Flex_Elem_1/1(Out1) -> Matrix Concatenate/1
  Flex_Elem_2/1(Out1) -> Matrix Concatenate/2
  Flex_Elem_3/1(Out1) -> Matrix Concatenate/3
  Flex_Elem_4/1(Out1) -> Matrix Concatenate/4
  Flex_Elem_5/1(Out1) -> Matrix Concatenate/5
  Flex_Elem_6/1(Out1) -> Matrix Concatenate/6
  Flex_Elem_7/1(Out1) -> Matrix Concatenate/7
  Flex_Elem_8/1(Out1) -> Matrix Concatenate/8
  Flex_Elem_9/1(Out1) -> Matrix Concatenate/9
  Flex_Elem_10/1(Out1) -> Matrix Concatenate/10
  Flex_Elem_11/1(Out1) -> Matrix Concatenate/11
  Flex_Elem_12/1(Out1) -> Matrix Concatenate/12
  Flex_Elem_13/1(Out1) -> Matrix Concatenate/13
  Flex_Elem_14/1(Out1) -> Matrix Concatenate/14
  Flex_Elem_15/1(Out1) -> Matrix Concatenate/15
  Flex_Elem_16/1(Out1) -> Matrix Concatenate/16
  Flex_Elem_17/1(Out1) -> Matrix Concatenate/17
  Flex_Elem_18/1(Out1) -> Matrix Concatenate/18
  Flex_Elem_19/1(Out1) -> Matrix Concatenate/19
  Flex_Elem_20/1(Out1) -> Matrix Concatenate/20
  Flex_Elem_21/1(Out1) -> Matrix Concatenate/21
  Flex_Elem_22/1(Out1) -> Matrix Concatenate/22
  Flex_Elem_23/1(Out1) -> Matrix Concatenate/23
  Flex_Elem_24/1(Out1) -> Matrix Concatenate/24
  Flex_Elem_25/1(Out1) -> Matrix Concatenate/25
  Flex_Elem_26/1(Out1) -> Matrix Concatenate/26
  Flex_Elem_27/1(Out1) -> Matrix Concatenate/27
  Flex_Elem_28/1(Out1) -> Matrix Concatenate/28
  Flex_Elem_29/1(Out1) -> Matrix Concatenate/29
  Flex_Elem_30/1(Out1) -> Matrix Concatenate/30
  Matrix Concatenate/1 -> Out1/1
  connections:
  B/RConn1 -- Transform BeamX/LConn1
  Transform BeamX/RConn1 -- Flex_Elem_1/LConn1
  Flex_Elem_1/RConn1 -- Flex_Elem_2/LConn1
  Flex_Elem_2/RConn1 -- Flex_Elem_3/LConn1
  Flex_Elem_3/RConn1 -- Flex_Elem_4/LConn1
  Flex_Elem_4/RConn1 -- Flex_Elem_5/LConn1
  Flex_Elem_5/RConn1 -- Flex_Elem_6/LConn1
  Flex_Elem_6/RConn1 -- Flex_Elem_7/LConn1
  Flex_Elem_7/RConn1 -- Flex_Elem_8/LConn1
  Flex_Elem_8/RConn1 -- Flex_Elem_9/LConn1
  Flex_Elem_9/RConn1 -- Flex_Elem_10/LConn1
  Flex_Elem_10/RConn1 -- Flex_Elem_11/LConn1
  Flex_Elem_11/RConn1 -- Flex_Elem_12/LConn1
  Flex_Elem_12/RConn1 -- Flex_Elem_13/LConn1
  Flex_Elem_13/RConn1 -- Flex_Elem_14/LConn1
  Flex_Elem_14/RConn1 -- Flex_Elem_15/LConn1
  Flex_Elem_15/RConn1 -- Flex_Elem_16/LConn1
  Flex_Elem_16/RConn1 -- Flex_Elem_17/LConn1
  Flex_Elem_17/RConn1 -- Flex_Elem_18/LConn1
  Flex_Elem_18/RConn1 -- Flex_Elem_19/LConn1
  Flex_Elem_19/RConn1 -- Flex_Elem_20/LConn1
  Flex_Elem_20/RConn1 -- Flex_Elem_21/LConn1
  Flex_Elem_21/RConn1 -- Flex_Elem_22/LConn1
  Flex_Elem_22/RConn1 -- Flex_Elem_23/LConn1
  Flex_Elem_23/RConn1 -- Flex_Elem_24/LConn1
  Flex_Elem_24/RConn1 -- Flex_Elem_25/LConn1
  Flex_Elem_25/RConn1 -- Flex_Elem_26/LConn1
  Flex_Elem_26/RConn1 -- Flex_Elem_27/LConn1
  Flex_Elem_27/RConn1 -- Flex_Elem_28/LConn1
  Flex_Elem_28/RConn1 -- Flex_Elem_29/LConn1
  Flex_Elem_29/RConn1 -- Flex_Elem_30/LConn1
  Flex_Elem_30/RConn1 -- F/RConn1

== system FlexBeamElement_MS2G_Lib/Flex_Element ==
  In1 : Inport
  Full : FlexBeamElement_MS2G_Lib/Full  length=length  rho=rho  beam_width=beam_width  beam_wall=beam_wall  kbendingx=kbendingx  kbendingy=kbendingy  kbendingz=ktwistz  kelongz=kelongz  b=b
  B : PMIOPort  Port=1  Side=Left
  F : PMIOPort  Port=2  Side=Right
  Out1 : Outport
  wires:
  In1/1 -> Full/1
  Full/1 -> Out1/1
  connections:
  Full/LConn1 -- B/RConn1
  Full/RConn1 -- F/RConn1
